simulink model "lyapunovControl"  (R2015a)
settings: Solver=ode3  StartTime=0.0  StopTime=26  FixedStep=0.001  RelTol=1e-3
values from neighbouring files (symbols this model uses):
  F = [1/r*1.1 L/r*1.1;1/r*1.1 -L/r*1.1]    [lyapunovInit.m]
  G = [r/2 r/2;r/(2*L) -r/(2*L)]    [lyapunovInit.m]
  R = 2    [lyapunovInit.m]
  theta0 = pi    (= 3.14159265359)    [lyapunovInit.m]
  wD = 0.5    [lyapunovInit.m]
  x0 = 2.3    [lyapunovInit.m]
  y0 = 0    [lyapunovInit.m]
undefined symbols (not defined in the file or in its folder): lyapu
libraries: simulink x2
settings Model: CovModelRefEnable=off  Creator=Subodh  LastModifiedBy=smishra
settings DataIOCC: SaveFormat=Dataset
settings HardwareCC: ProdBitPerPointer=64  ProdLargestAtomicFloat=Float  ProdIntDivRoundTo=Zero  ProdEndianess=LittleEndian  ProdHWDeviceType=Specified
settings GRTTargetCC: GeneratePreprocessorConditionals=Use local settings

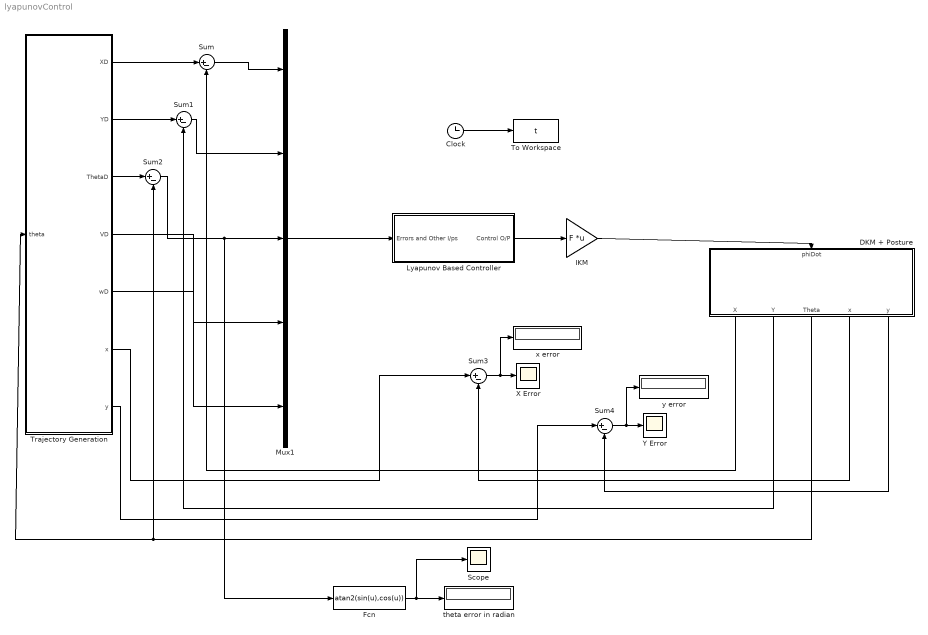
== system lyapunovControl ==
  Clock : Clock
  DKM + Posture : Subsystem
  Fcn : Fcn  Expr=atan2(sin(u),cos(u))
  IKM : Gain  Gain=F  Multiplication=Matrix(K*u)
  Lyapunov Based Controller : Subsystem
  Mux1 : Mux  Inputs=5
  Scope : Scope
      settings: YMin=-1.76715  YMax=0.19635
  Sum{,1..4} (5 alike) : Sum  Inputs=|+-
  To Workspace : ToWorkspace  VariableName=t  SampleTime=-1
  Trajectory Generation : Subsystem
  X Error : Scope
      settings: YMin=-0.33752  YMax=0.03768
  Y Error : Scope
      settings: YMin=-0.11626  YMax=0.08605  SaveName=ScopeData2
  theta error in radian : Display
  "x error " : Display
  y error : Display
  wires:
  IKM/1 -> DKM + Posture/1(phiDot)
  Trajectory Generation/1(XD) -> Sum/1
  Trajectory Generation/2(YD) -> Sum1/1
  Trajectory Generation/3(ThetaD) -> Sum2/1
  DKM + Posture/1(X) -> Sum/2
  DKM + Posture/2(Y) -> Sum1/2
  DKM + Posture/3(Theta) -> Trajectory Generation/1(theta), Sum2/2
  Sum1/1 -> Mux1/2
  Sum/1 -> Mux1/1
  Sum2/1 -> Fcn/1, Mux1/3
  Trajectory Generation/4(VD) -> Mux1/4
  Trajectory Generation/5(wD) -> Mux1/5
  Mux1/1 -> Lyapunov Based Controller/1(Errors and Other I/ps)
  Lyapunov Based Controller/1(Control O/P) -> IKM/1
  Fcn/1 -> Scope/1, theta error in radian/1
  Trajectory Generation/6(x) -> Sum3/1
  DKM + Posture/4(x) -> Sum3/2
  Sum3/1 -> "x error "/1, X Error/1
  Sum4/1 -> y error/1, Y Error/1
  DKM + Posture/5(y) -> Sum4/2
  Trajectory Generation/7(y) -> Sum4/1
  Clock/1 -> To Workspace/1

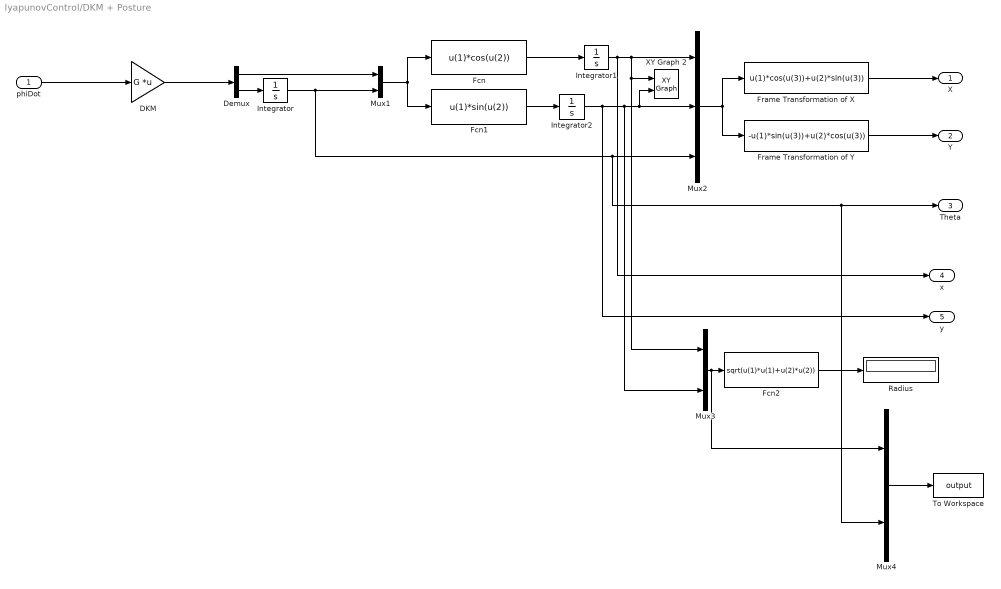
== system lyapunovControl/DKM + Posture ==
  phiDot : Inport
  DKM : Gain  Gain=G  Multiplication=Matrix(K*u)
  Demux : Demux  Outputs=2
  Fcn : Fcn  Expr=u(1)*cos(u(2))
  Fcn1 : Fcn  Expr=u(1)*sin(u(2))
  Fcn2 : Fcn  Expr=sqrt(u(1)*u(1)+u(2)*u(2))
  Frame Transformation of X : Fcn  Expr=u(1)*cos(u(3))+u(2)*sin(u(3))
  Frame Transformation of Y : Fcn  Expr=-u(1)*sin(u(3))+u(2)*cos(u(3))
  Integrator : Integrator  InitialCondition=theta0
  Integrator1 : Integrator  InitialCondition=x0
  Integrator2 : Integrator  InitialCondition=y0
  Mux1 : Mux  Inputs=2
  Mux2 : Mux  Inputs=3
  Mux3 : Mux  Inputs=2
  Mux4 : Mux  Inputs=2
  Radius : Display
  To Workspace : ToWorkspace  VariableName=output  SampleTime=-1
  XY Graph 2 : simulink/Sinks/XY Graph  xmin=-2.3  xmax=2.3  ymin=-2.3  ymax=2.3  st=-1
  X : Outport
  Y : Outport  Port=2
  Theta : Outport  Port=3
  x : Outport  Port=4
  y : Outport  Port=5
  wires:
  DKM/1 -> Demux/1
  Demux/1 -> Mux1/1
  phiDot/1 -> DKM/1
  Demux/2 -> Integrator/1
  Mux1/1 -> Fcn1/1, Fcn/1
  Fcn/1 -> Integrator1/1
  Fcn1/1 -> Integrator2/1
  Frame Transformation of X/1 -> X/1
  Frame Transformation of Y/1 -> Y/1
  Integrator1/1 -> x/1, Mux3/1, XY Graph 2/1, Mux2/1
  Mux2/1 -> Frame Transformation of X/1, Frame Transformation of Y/1
  Integrator/1 -> Mux4/2, Theta/1, Mux2/3, Mux1/2
  Mux3/1 -> Mux4/1, Fcn2/1
  Fcn2/1 -> Radius/1
  Mux4/1 -> To Workspace/1
  Integrator2/1 -> y/1, Mux3/2, XY Graph 2/2, Mux2/2

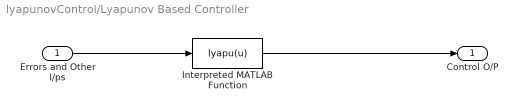
== system lyapunovControl/Lyapunov Based Controller ==
  Errors and Other I/ps : Inport
  Interpreted MATLAB Function : MATLABFcn  MATLABFcn=lyapu(u)  OutputDimensions=2
  Control O/P : Outport
  wires:
  Interpreted MATLAB Function/1 -> Control O/P/1
  Errors and Other I/ps/1 -> Interpreted MATLAB Function/1

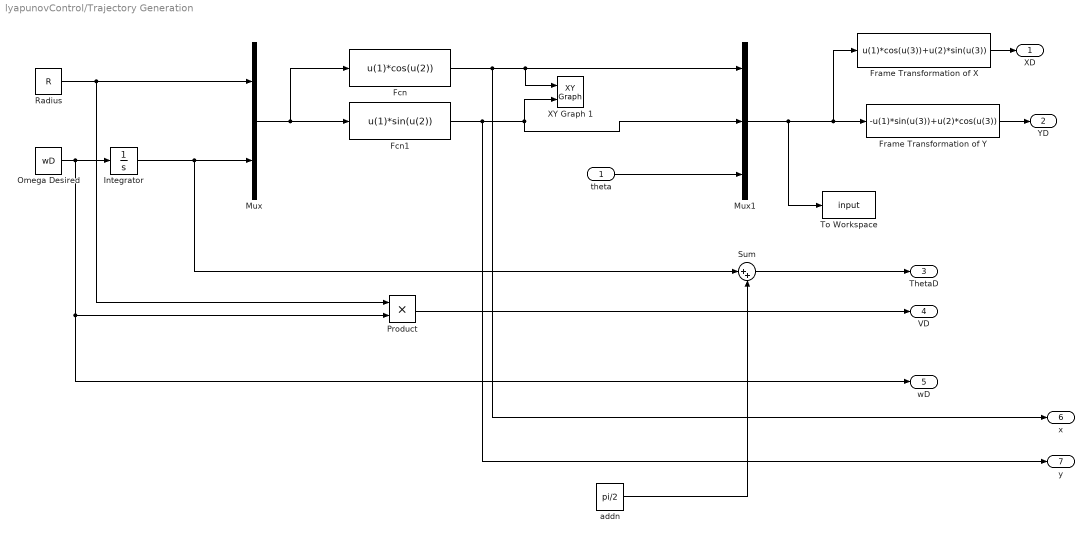
== system lyapunovControl/Trajectory Generation ==
  theta : Inport
  Fcn : Fcn  Expr=u(1)*cos(u(2))
  Fcn1 : Fcn  Expr=u(1)*sin(u(2))
  Frame Transformation of X : Fcn  Expr=u(1)*cos(u(3))+u(2)*sin(u(3))
  Frame Transformation of Y : Fcn  Expr=-u(1)*sin(u(3))+u(2)*cos(u(3))
  Integrator : Integrator
  Mux : Mux  Inputs=2
  Mux1 : Mux  Inputs=3
  Omega Desired : Constant  Value=wD
  Product : Product
  Radius : Constant  Value=R
  Sum : Sum  Inputs=|++
  To Workspace : ToWorkspace  VariableName=input  SampleTime=-1
  XY Graph 1 : simulink/Sinks/XY Graph  xmin=-2.3  xmax=2.3  ymin=-2.3  ymax=2.3  st=-1
  addn : Constant  Value=pi/2
  XD : Outport
  YD : Outport  Port=2
  ThetaD : Outport  Port=3
  VD : Outport  Port=4
  wD : Outport  Port=5
  x : Outport  Port=6
  y : Outport  Port=7
  wires:
  Fcn1/1 -> y/1, XY Graph 1/2, Mux1/2
  Fcn/1 -> x/1, Mux1/1, XY Graph 1/1
  Product/1 -> VD/1
  Radius/1 -> Mux/1, Product/1
  Omega Desired/1 -> Integrator/1, Product/2, wD/1
  Mux/1 -> Fcn1/1, Fcn/1
  Integrator/1 -> Sum/1, Mux/2
  theta/1 -> Mux1/3
  Frame Transformation of X/1 -> XD/1
  Mux1/1 -> To Workspace/1, Frame Transformation of X/1, Frame Transformation of Y/1
  Frame Transformation of Y/1 -> YD/1
  Sum/1 -> ThetaD/1
  addn/1 -> Sum/2
